simulink model "SSN_39busRT_Ctrl_4WT_19B"  (R2021a)
settings: Solver=ode3  StartTime=0.0  StopTime=10  FixedStep=Ts  MaxStep=1/60  RelTol=1e-2  AbsTol=1e-1
PreLoadFcn:
  | Ts=2.50e-6; ssn_ieee39_params; load('Pwf.mat');
InitFcn:
  | Ts=2.50e-6; ssn_ieee39_params; load('Pwf.mat');
values from neighbouring files (symbols this model uses):
  f = 50    [ssn_ieee39_params_ctrl.m]
  fNom = f    (= 60)    [ssn_ieee39_params_ctrl.m]
  ILR = 5.02    [ssn_ieee39_params_ctrl.m]
  IQMIN = 0.1    [ssn_ieee39_params_ctrl.m]
  ISCLIM = 1    [ssn_ieee39_params_ctrl.m]
  ITFpu = 1.10    (= 1.1)    [ssn_ieee39_params_ctrl.m]
  K = 1    [ssn_ieee39_params_ctrl.m]
  K1 = 1    [ssn_ieee39_params_ctrl.m]
  K2 = 2    [ssn_ieee39_params_ctrl.m]
  KCL = 1.04    [ssn_ieee39_params_ctrl.m]
  KFB = 0    [ssn_ieee39_params_ctrl.m]
  KFF = 1    [ssn_ieee39_params_ctrl.m]
  KFIX = 1    [ssn_ieee39_params_ctrl.m]
  KG = 1    [ssn_ieee39_params_ctrl.m]
  KIA = 59.91    [ssn_ieee39_params_ctrl.m]
  KIOEX = 0.0303    [ssn_ieee39_params_ctrl.m]
  KIUEX = 0.0303    [ssn_ieee39_params_ctrl.m]
  KIUOEX = 1    [ssn_ieee39_params_ctrl.m]
  KIUUEX = 1    [ssn_ieee39_params_ctrl.m]
  KLR = 22.47    [ssn_ieee39_params_ctrl.m]
  KM = 1    [ssn_ieee39_params_ctrl.m]
  KOEL = 0.24    [ssn_ieee39_params_ctrl.m]
  Kp = 1    [ssn_ieee39_params_ctrl.m]
  KPA = 30    [ssn_ieee39_params_ctrl.m]
  KPOEL = 1    [ssn_ieee39_params_ctrl.m]
  KPOEX = 0    [ssn_ieee39_params_ctrl.m]
  KPUEX = 0    [ssn_ieee39_params_ctrl.m]
  KSCALE = 0.319    [ssn_ieee39_params_ctrl.m]
  KUF = 0    [ssn_ieee39_params_ctrl.m]
  KUI = 0.001    [ssn_ieee39_params_ctrl.m]
  KUL = 0.24    [ssn_ieee39_params_ctrl.m]
  s = 10    [ssn_ieee39_params_ctrl.m]
  TA = 0.01    [ssn_ieee39_params_ctrl.m]
  Tadj = 0    [ssn_ieee39_params_ctrl.m]
  taps = [1 1 1.07 1.07 1.009 1.025 1 1.025 1.025 1.025]*1    [ssn_ieee39_params_ctrl.m]
  TF = 0.02    [ssn_ieee39_params_ctrl.m]
  TG = 0.024    [ssn_ieee39_params_ctrl.m]
  TINV = 0    [ssn_ieee39_params_ctrl.m]
  TIT = 0.1    [ssn_ieee39_params_ctrl.m]
  TL_10_11_len = 14    [ssn_ieee39_params_ctrl.m]
  TL_10_13_len = 14    [ssn_ieee39_params_ctrl.m]
  TL_13_14_len = 32    [ssn_ieee39_params_ctrl.m]
  TL_14_15_len = 70    [ssn_ieee39_params_ctrl.m]
  TL_15_16_len = 31.5    [ssn_ieee39_params_ctrl.m]
  TL_16_17_len = 26    [ssn_ieee39_params_ctrl.m]
  TL_16_19_len = 61    [ssn_ieee39_params_ctrl.m]
  TL_16_21_len = 46    [ssn_ieee39_params_ctrl.m]
  TL_16_24_len = 15    [ssn_ieee39_params_ctrl.m]
  TL_17_18_len = 26    [ssn_ieee39_params_ctrl.m]
  TL_17_27_len = 59    [ssn_ieee39_params_ctrl.m]
  TL_1_2_len = 134    [ssn_ieee39_params_ctrl.m]
  TL_1_39_len = 105    [ssn_ieee39_params_ctrl.m]
  TL_21_22_len = 47    [ssn_ieee39_params_ctrl.m]
  TL_22_23_len = 33    [ssn_ieee39_params_ctrl.m]
  TL_24_23_len = 88    [ssn_ieee39_params_ctrl.m]
  TL_25_26_len = 101    [ssn_ieee39_params_ctrl.m]
  TL_26_27_len = 46.5    [ssn_ieee39_params_ctrl.m]
  TL_26_28_len = 151    [ssn_ieee39_params_ctrl.m]
  TL_26_29_len = 200    [ssn_ieee39_params_ctrl.m]
  TL_28_29_len = 48    [ssn_ieee39_params_ctrl.m]
  TL_2_25_len = 28    [ssn_ieee39_params_ctrl.m]
  TL_2_2_len = 49    [ssn_ieee39_params_ctrl.m]
  TL_3_18_len = 42    [ssn_ieee39_params_ctrl.m]
  TL_3_4_len = 53    [ssn_ieee39_params_ctrl.m]
  TL_4_14_len = 33    [ssn_ieee39_params_ctrl.m]
  TL_4_5_len = 32.5    [ssn_ieee39_params_ctrl.m]
  TL_5_6_len = 14    [ssn_ieee39_params_ctrl.m]
  TL_5_8_len = 32    [ssn_ieee39_params_ctrl.m]
  TL_6_11_len = 26.5    [ssn_ieee39_params_ctrl.m]
  TL_6_7_len = 25.5    [ssn_ieee39_params_ctrl.m]
  TL_7_8_len = 15    [ssn_ieee39_params_ctrl.m]
  TL_8_9_len = 93    [ssn_ieee39_params_ctrl.m]
  TL_9_39_len = 136    [ssn_ieee39_params_ctrl.m]
  TOEL = 5.00    (= 5)    [ssn_ieee39_params_ctrl.m]
  TQREF = 0    [ssn_ieee39_params_ctrl.m]
  TQSCL = 0.012    [ssn_ieee39_params_ctrl.m]
  Ts_PMU = 1/1000    (= 0.001)    [ssn_ieee39_params_ctrl.m]
  TU1 = 0    [ssn_ieee39_params_ctrl.m]
  TU2 = 0    [ssn_ieee39_params_ctrl.m]
  TU3 = 0    [ssn_ieee39_params_ctrl.m]
  TU4 = 0    [ssn_ieee39_params_ctrl.m]
  TUL = 0    [ssn_ieee39_params_ctrl.m]
  TUP = 0.050    (= 0.05)    [ssn_ieee39_params_ctrl.m]
  TUQ = .005    (= 0.005)    [ssn_ieee39_params_ctrl.m]
  TUV = 0.2    [ssn_ieee39_params_ctrl.m]
  VAAMAX = VAMAX    (= 7.05)    [ssn_ieee39_params_ctrl.m]
  VAMAX = 7.05    [ssn_ieee39_params_ctrl.m]
  VAMIN = -6.11    [ssn_ieee39_params_ctrl.m]
  VBMAX = 999    [ssn_ieee39_params_ctrl.m]
  VF = 0    [ssn_ieee39_params_ctrl.m]
  VFB = 0    [ssn_ieee39_params_ctrl.m]
  VMMAX = 7.05    [ssn_ieee39_params_ctrl.m]
  VMMIN = -6.11    [ssn_ieee39_params_ctrl.m]
  VOELmax1 = 0.2353    [ssn_ieee39_params_ctrl.m]
  VOELmax2 = 0.0    (= 0)    [ssn_ieee39_params_ctrl.m]
  VOELmin1 = -0.24    [ssn_ieee39_params_ctrl.m]
  VOELmin2 = -1.0    (= -1)    [ssn_ieee39_params_ctrl.m]
  VRMAX = 7.05    [ssn_ieee39_params_ctrl.m]
  VRMIN = -6.11    [ssn_ieee39_params_ctrl.m]
  VSCLmax = 0.20    (= 0.2)    [ssn_ieee39_params_ctrl.m]
  VSCLmin = -0.10    (= -0.1)    [ssn_ieee39_params_ctrl.m]
  VUELmax1 = 1    [ssn_ieee39_params_ctrl.m]
  VUELmax2 = 1    [ssn_ieee39_params_ctrl.m]
  VUELmin1 = -1    [ssn_ieee39_params_ctrl.m]
  VUELmin2 = -1    [ssn_ieee39_params_ctrl.m]
  VUImax = 1    [ssn_ieee39_params_ctrl.m]
  VUImin = -1    [ssn_ieee39_params_ctrl.m]
undefined symbols (not defined in the file or in its folder): another_event_name, D1, Delta, DiscIntNeverNeededParam, find_system, MOV_segment9, my_event_name, powergui, Pw1, Pw2, Pw3, Pw4, vNomHV
libraries: powerlib_extras x162, spsThreePhaseVIMeasurementLib x55, spsCurrentMeasurementLib x52, simulink_extras x44, slpidlib x40, op_dpl_lib x36, spsST2AModel x20, spsThreePhaseParallelRLCLoadLib x20, spsThreePhaseTransformerTwoWindingsLib x17, spsControlledVoltageSourceLib x16, spsVoltageMeasurementLib x12, spsSynchronousMachinepuStandardLib x10
(part 4 of 19)

== system SSN_39busRT_Ctrl_4WT_19B/SM_master/PMU_Vpos_60Hz7 ==
  abc : Inport  PortDimensions=3
  1 / sqrt of 2 : Gain  Gain=1/sqrt(2)  OutDataTypeStr=Inherit: Same as input  ParamDataTypeStr=Inherit: Same as input
  Cartesian to Polar : simulink_extras/Transformations/Cartesian to Polar
  Demux : Demux  Outputs=3
      settings: DisplayOption=none
  Discrete Mean value1 : powerlib_extras/Discrete Measurements/Discrete  Mean value  Freq=Freq  Vinit=Real_Init  Ts=Ts
      settings: SourceProductBaseCode=PS
  Discrete Mean value2 : powerlib_extras/Discrete Measurements/Discrete  Mean value  Freq=Freq  Vinit=Imag_Init  Ts=Ts
      settings: SourceProductBaseCode=PS
  Discrete Derivative : simulink/Discrete/Discrete Derivative  gainval=1.0  ICPrevScaledInput=0.0  OutMin=[]  OutMax=[]  OutDataType=fixdt(1, 16)  OutScaling=2^-10  DoSatur=off
  Gain : Gain  Gain=2*pi*Freq  SaturateOnIntegerOverflow=on  OutDataTypeStr=Inherit: Same as input  ParamDataTypeStr=Inherit: Same as input
  Mux : Mux  Inputs=2
  Rad->Deg. : Gain  Gain=180/pi  SaturateOnIntegerOverflow=on  OutDataTypeStr=Inherit: Same as input  ParamDataTypeStr=Inherit: Same as input
  Sum : Sum  Inputs=|++  OutDataTypeStr=Inherit: Same as first input
  Terminator : Terminator
  Trigonometric Function : Trigonometry
  Trigonometric Function1 : Trigonometry  Operator=cos
  abc_to_dq0 Transformation : powerlib_extras/Measurements/abc_to_dq0 Transformation
      settings: SourceProductBaseCode=PS
  fo : Constant  Value=2*pi*Freq
  t : DigitalClock  SampleTime=Ts
  Mag : Outport
  Phase : Outport  Port=2
  freq : Outport  Port=3
  dfdt : Outport  Port=4
  wires:
  Cartesian to Polar/2 -> Rad->Deg./1, Discrete Derivative/1
  Gain/1 -> Trigonometric Function1/1, Trigonometric Function/1
  t/1 -> Gain/1
  abc/1 -> abc_to_dq0 Transformation/1
  Mux/1 -> abc_to_dq0 Transformation/2
  Discrete Mean value1/1 -> Cartesian to Polar/1  "Real"
  Rad->Deg./1 -> Phase/1
  Discrete Mean value2/1 -> Cartesian to Polar/2  "Real"
  abc_to_dq0 Transformation/1 -> Demux/1
  Demux/3 -> Terminator/1
  Demux/2 -> Discrete Mean value2/1
  Demux/1 -> Discrete Mean value1/1
  Trigonometric Function/1 -> Mux/1
  Trigonometric Function1/1 -> Mux/2
  Cartesian to Polar/1 -> 1 / sqrt of 2/1
  1 / sqrt of 2/1 -> Mag/1
  Discrete Derivative/1 -> Sum/2, dfdt/1
  fo/1 -> Sum/1
  Sum/1 -> freq/1

== system SSN_39busRT_Ctrl_4WT_19B/SM_master/PMU_Vpos_60Hz8 ==
  abc : Inport  PortDimensions=3
  1 / sqrt of 2 : Gain  Gain=1/sqrt(2)  OutDataTypeStr=Inherit: Same as input  ParamDataTypeStr=Inherit: Same as input
  Cartesian to Polar : simulink_extras/Transformations/Cartesian to Polar
  Demux : Demux  Outputs=3
      settings: DisplayOption=none
  Discrete Mean value1 : powerlib_extras/Discrete Measurements/Discrete  Mean value  Freq=Freq  Vinit=Real_Init  Ts=Ts
      settings: SourceProductBaseCode=PS
  Discrete Mean value2 : powerlib_extras/Discrete Measurements/Discrete  Mean value  Freq=Freq  Vinit=Imag_Init  Ts=Ts
      settings: SourceProductBaseCode=PS
  Discrete Derivative : simulink/Discrete/Discrete Derivative  gainval=1.0  ICPrevScaledInput=0.0  OutMin=[]  OutMax=[]  OutDataType=fixdt(1, 16)  OutScaling=2^-10  DoSatur=off
  Gain : Gain  Gain=2*pi*Freq  SaturateOnIntegerOverflow=on  OutDataTypeStr=Inherit: Same as input  ParamDataTypeStr=Inherit: Same as input
  Mux : Mux  Inputs=2
  Rad->Deg. : Gain  Gain=180/pi  SaturateOnIntegerOverflow=on  OutDataTypeStr=Inherit: Same as input  ParamDataTypeStr=Inherit: Same as input
  Sum : Sum  Inputs=|++  OutDataTypeStr=Inherit: Same as first input
  Terminator : Terminator
  Trigonometric Function : Trigonometry
  Trigonometric Function1 : Trigonometry  Operator=cos
  abc_to_dq0 Transformation : powerlib_extras/Measurements/abc_to_dq0 Transformation
      settings: SourceProductBaseCode=PS
  fo : Constant  Value=2*pi*Freq
  t : DigitalClock  SampleTime=Ts
  Mag : Outport
  Phase : Outport  Port=2
  freq : Outport  Port=3
  dfdt : Outport  Port=4
  wires:
  Cartesian to Polar/2 -> Rad->Deg./1, Discrete Derivative/1
  Gain/1 -> Trigonometric Function1/1, Trigonometric Function/1
  t/1 -> Gain/1
  abc/1 -> abc_to_dq0 Transformation/1
  Mux/1 -> abc_to_dq0 Transformation/2
  Discrete Mean value1/1 -> Cartesian to Polar/1  "Real"
  Rad->Deg./1 -> Phase/1
  Discrete Mean value2/1 -> Cartesian to Polar/2  "Real"
  abc_to_dq0 Transformation/1 -> Demux/1
  Demux/3 -> Terminator/1
  Demux/2 -> Discrete Mean value2/1
  Demux/1 -> Discrete Mean value1/1
  Trigonometric Function/1 -> Mux/1
  Trigonometric Function1/1 -> Mux/2
  Cartesian to Polar/1 -> 1 / sqrt of 2/1
  1 / sqrt of 2/1 -> Mag/1
  Discrete Derivative/1 -> Sum/2, dfdt/1
  fo/1 -> Sum/1
  Sum/1 -> freq/1

== system SSN_39busRT_Ctrl_4WT_19B/SM_master/PMU_Vpos_60Hz9 ==
  abc : Inport  PortDimensions=3
  1 / sqrt of 2 : Gain  Gain=1/sqrt(2)  OutDataTypeStr=Inherit: Same as input  ParamDataTypeStr=Inherit: Same as input
  Cartesian to Polar : simulink_extras/Transformations/Cartesian to Polar
  Demux : Demux  Outputs=3
      settings: DisplayOption=none
  Discrete Mean value1 : powerlib_extras/Discrete Measurements/Discrete  Mean value  Freq=Freq  Vinit=Real_Init  Ts=Ts
      settings: SourceProductBaseCode=PS
  Discrete Mean value2 : powerlib_extras/Discrete Measurements/Discrete  Mean value  Freq=Freq  Vinit=Imag_Init  Ts=Ts
      settings: SourceProductBaseCode=PS
  Discrete Derivative : simulink/Discrete/Discrete Derivative  gainval=1.0  ICPrevScaledInput=0.0  OutMin=[]  OutMax=[]  OutDataType=fixdt(1, 16)  OutScaling=2^-10  DoSatur=off
  Gain : Gain  Gain=2*pi*Freq  SaturateOnIntegerOverflow=on  OutDataTypeStr=Inherit: Same as input  ParamDataTypeStr=Inherit: Same as input
  Mux : Mux  Inputs=2
  Rad->Deg. : Gain  Gain=180/pi  SaturateOnIntegerOverflow=on  OutDataTypeStr=Inherit: Same as input  ParamDataTypeStr=Inherit: Same as input
  Sum : Sum  Inputs=|++  OutDataTypeStr=Inherit: Same as first input
  Terminator : Terminator
  Trigonometric Function : Trigonometry
  Trigonometric Function1 : Trigonometry  Operator=cos
  abc_to_dq0 Transformation : powerlib_extras/Measurements/abc_to_dq0 Transformation
      settings: SourceProductBaseCode=PS
  fo : Constant  Value=2*pi*Freq
  t : DigitalClock  SampleTime=Ts
  Mag : Outport
  Phase : Outport  Port=2
  freq : Outport  Port=3
  dfdt : Outport  Port=4
  wires:
  Cartesian to Polar/2 -> Rad->Deg./1, Discrete Derivative/1
  Gain/1 -> Trigonometric Function1/1, Trigonometric Function/1
  t/1 -> Gain/1
  abc/1 -> abc_to_dq0 Transformation/1
  Mux/1 -> abc_to_dq0 Transformation/2
  Discrete Mean value1/1 -> Cartesian to Polar/1  "Real"
  Rad->Deg./1 -> Phase/1
  Discrete Mean value2/1 -> Cartesian to Polar/2  "Real"
  abc_to_dq0 Transformation/1 -> Demux/1
  Demux/3 -> Terminator/1
  Demux/2 -> Discrete Mean value2/1
  Demux/1 -> Discrete Mean value1/1
  Trigonometric Function/1 -> Mux/1
  Trigonometric Function1/1 -> Mux/2
  Cartesian to Polar/1 -> 1 / sqrt of 2/1
  1 / sqrt of 2/1 -> Mag/1
  Discrete Derivative/1 -> Sum/2, dfdt/1
  fo/1 -> Sum/1
  Sum/1 -> freq/1

== system SSN_39busRT_Ctrl_4WT_19B/SM_master/Power ==
  Mux : Mux  Inputs=10
  Power (3ph, Instantaneous){1..10} (10 alike) : spsPower3phInstantaneousLib/Power (3ph, Instantaneous)
  Scope{1..10} (10 alike) : Scope  NumInputPorts=2
  to PU{1..20} (20 alike) : Gain
  Pgen : Outport
  tag scope: PG_10=global, PG_1=global, PG_2=global, PG_3=global, PG_4=global, PG_5=global, PG_6=global, PG_7=global, PG_8=global, PG_9=global
  wires:
  [Iabc_30] -> "Power (3ph, Instantaneous)1"/2
  to PU2/1 -> Scope7/2, [QG_10]
  [Vabc_30] -> "Power (3ph, Instantaneous)1"/1
  "Power (3ph, Instantaneous)4"/2 -> to PU9/1
  to PU8/1 -> [PG_8], Scope4/1
  "Power (3ph, Instantaneous)1"/1 -> to PU1/1
  "Power (3ph, Instantaneous)1"/2 -> to PU2/1
  "Power (3ph, Instantaneous)4"/1 -> to PU8/1
  [Vabc_37] -> "Power (3ph, Instantaneous)4"/1
  to PU1/1 -> Scope7/1, [PG_10]
  [Iabc_37] -> "Power (3ph, Instantaneous)4"/2
  to PU9/1 -> [QG_8], Scope4/2
  to PU6/1 -> Scope1/2, [QG_9]
  [Iabc_38] -> "Power (3ph, Instantaneous)3"/2
  to PU3/1 -> [PG_1], Scope2/1
  [Vabc_38] -> "Power (3ph, Instantaneous)3"/1
  "Power (3ph, Instantaneous)3"/1 -> to PU5/1
  "Power (3ph, Instantaneous)2"/2 -> to PU4/1
  "Power (3ph, Instantaneous)2"/1 -> to PU3/1
  to PU5/1 -> Scope1/1, [PG_9]
  "Power (3ph, Instantaneous)3"/2 -> to PU6/1
  [Vabc_391] -> "Power (3ph, Instantaneous)2"/1
  to PU4/1 -> [QG_1], Scope2/2
  [Iabc_391] -> "Power (3ph, Instantaneous)2"/2
  [Iabc_34] -> "Power (3ph, Instantaneous)6"/2
  to PU12/1 -> Scope5/2, [QG_5]
  [Vabc_34] -> "Power (3ph, Instantaneous)6"/1
  "Power (3ph, Instantaneous)7"/2 -> to PU14/1
  to PU13/1 -> [PG_4], Scope3/1
  "Power (3ph, Instantaneous)6"/1 -> to PU11/1
  "Power (3ph, Instantaneous)6"/2 -> to PU12/1
  "Power (3ph, Instantaneous)7"/1 -> to PU13/1
  [Vabc_33] -> "Power (3ph, Instantaneous)7"/1
  to PU11/1 -> Scope5/1, [PG_5]
  [Iabc_33] -> "Power (3ph, Instantaneous)7"/2
  to PU14/1 -> [QG_4], Scope3/2
  to PU16/1 -> Scope6/2, [QG_2]
  [Iabc_31] -> "Power (3ph, Instantaneous)8"/2
  to PU7/1 -> [PG_3], Scope8/1
  [Vabc_31] -> "Power (3ph, Instantaneous)8"/1
  "Power (3ph, Instantaneous)8"/1 -> to PU15/1
  "Power (3ph, Instantaneous)5"/2 -> to PU10/1
  "Power (3ph, Instantaneous)5"/1 -> to PU7/1
  to PU15/1 -> Scope6/1, [PG_2]
  "Power (3ph, Instantaneous)8"/2 -> to PU16/1
  [Vabc_32] -> "Power (3ph, Instantaneous)5"/1
  to PU10/1 -> [QG_3], Scope8/2
  [Iabc_32] -> "Power (3ph, Instantaneous)5"/2
  [Iabc_35] -> "Power (3ph, Instantaneous)9"/2
  to PU17/1 -> Scope10/2, [QG_6]
  [Vabc_35] -> "Power (3ph, Instantaneous)9"/1
  "Power (3ph, Instantaneous)9"/1 -> to PU20/1
  "Power (3ph, Instantaneous)9"/2 -> to PU17/1
  to PU20/1 -> Scope10/1, [PG_6]
  to PU18/1 -> [PG_7], Scope9/1
  "Power (3ph, Instantaneous)10"/2 -> to PU19/1
  "Power (3ph, Instantaneous)10"/1 -> to PU18/1
  [Vabc_36] -> "Power (3ph, Instantaneous)10"/1
  to PU19/1 -> [QG_7], Scope9/2
  [Iabc_36] -> "Power (3ph, Instantaneous)10"/2
  [PG_1] -> Mux/1
  [PG_2] -> Mux/2
  [PG_3] -> Mux/3
  [PG_4] -> Mux/4
  [PG_5] -> Mux/5
  [PG_6] -> Mux/6
  [PG_7] -> Mux/7
  [PG_8] -> Mux/8
  [PG_9] -> Mux/9
  [PG_10] -> Mux/10
  Mux/1 -> Pgen/1

== system SSN_39busRT_Ctrl_4WT_19B/powergui/EquivalentModel1 ==
  Sources : Subsystem
  State-Space : S-Function  FunctionName=ssn_sfun_v1  Parameters=1,0  SFunctionDeploymentMode=off  EnableBusSupport=off  SFcnStateName=MOV_segment9,MOV_segment9,MOV_segment9,MOV_segment9,MOV_segment9,MOV_segment9,MOV_segment9,MOV_segment9,MOV_segment9,MOV_segment9
      settings: SFcnIsStateOwnerBlock=on
  Yout : Subsystem
  wires:
  State-Space/1 -> Yout/1(v,i)
  Sources/1(u) -> State-Space/1

== system SSN_39busRT_Ctrl_4WT_19B/powergui/EquivalentModel10 ==
  Sources : Subsystem
  State-Space : S-Function  FunctionName=ssn_sfun_v1  Parameters=10,0  SFunctionDeploymentMode=off  EnableBusSupport=off  SFcnStateName=MOV_segment9,MOV_segment9,MOV_segment9,MOV_segment9,MOV_segment9,MOV_segment9,MOV_segment9,MOV_segment9,MOV_segment9,MOV_segment9
      settings: SFcnIsStateOwnerBlock=on
  Yout : Subsystem
  wires:
  State-Space/1 -> Yout/1(v,i)
  Sources/1(u) -> State-Space/1

== system SSN_39busRT_Ctrl_4WT_19B/powergui/EquivalentModel11 ==
  Sources : Subsystem
  State-Space : S-Function  FunctionName=ssn_sfun_v1  Parameters=11,0  SFunctionDeploymentMode=off  EnableBusSupport=off  SFcnStateName=MOV_segment9,MOV_segment9,MOV_segment9,MOV_segment9,MOV_segment9,MOV_segment9,MOV_segment9,MOV_segment9,MOV_segment9,MOV_segment9
      settings: SFcnIsStateOwnerBlock=on
  Yout : Subsystem
  wires:
  State-Space/1 -> Yout/1(v,i)
  Sources/1(u) -> State-Space/1

== system SSN_39busRT_Ctrl_4WT_19B/powergui/EquivalentModel12 ==
  Sources : Subsystem
  State-Space : S-Function  FunctionName=ssn_sfun_v1  Parameters=12,0  SFunctionDeploymentMode=off  EnableBusSupport=off  SFcnStateName=MOV_segment9,MOV_segment9,MOV_segment9,MOV_segment9,MOV_segment9,MOV_segment9,MOV_segment9,MOV_segment9,MOV_segment9,MOV_segment9
      settings: SFcnIsStateOwnerBlock=on
  Yout : Subsystem
  wires:
  State-Space/1 -> Yout/1(v,i)
  Sources/1(u) -> State-Space/1

== system SSN_39busRT_Ctrl_4WT_19B/powergui/EquivalentModel13 ==
  Sources : Subsystem
  State-Space : S-Function  FunctionName=ssn_sfun_v1  Parameters=13,0  SFunctionDeploymentMode=off  EnableBusSupport=off  SFcnStateName=MOV_segment9,MOV_segment9,MOV_segment9,MOV_segment9,MOV_segment9,MOV_segment9,MOV_segment9,MOV_segment9,MOV_segment9,MOV_segment9
      settings: SFcnIsStateOwnerBlock=on
  Yout : Subsystem
  wires:
  State-Space/1 -> Yout/1(v,i)
  Sources/1(u) -> State-Space/1

== system SSN_39busRT_Ctrl_4WT_19B/powergui/EquivalentModel14 ==
  Sources : Subsystem
  State-Space : S-Function  FunctionName=ssn_sfun_v1  Parameters=14,0  SFunctionDeploymentMode=off  EnableBusSupport=off  SFcnStateName=MOV_segment9,MOV_segment9,MOV_segment9,MOV_segment9,MOV_segment9,MOV_segment9,MOV_segment9,MOV_segment9,MOV_segment9,MOV_segment9
      settings: SFcnIsStateOwnerBlock=on
  Yout : Subsystem
  wires:
  State-Space/1 -> Yout/1(v,i)
  Sources/1(u) -> State-Space/1

== system SSN_39busRT_Ctrl_4WT_19B/powergui/EquivalentModel15 ==
  Sources : Subsystem
  State-Space : S-Function  FunctionName=ssn_sfun_v1  Parameters=15,0  SFunctionDeploymentMode=off  EnableBusSupport=off  SFcnStateName=MOV_segment9,MOV_segment9,MOV_segment9,MOV_segment9,MOV_segment9,MOV_segment9,MOV_segment9,MOV_segment9,MOV_segment9,MOV_segment9
      settings: SFcnIsStateOwnerBlock=on
  Yout : Subsystem
  wires:
  State-Space/1 -> Yout/1(v,i)
  Sources/1(u) -> State-Space/1

== system SSN_39busRT_Ctrl_4WT_19B/powergui/EquivalentModel16 ==
  Gates : Subsystem
  Sources : Subsystem
  State-Space : S-Function  FunctionName=ssn_sfun_v1  Parameters=16,0  SFunctionDeploymentMode=off  EnableBusSupport=off  SFcnStateName=MOV_segment9,MOV_segment9,MOV_segment9,MOV_segment9,MOV_segment9,MOV_segment9,MOV_segment9,MOV_segment9,MOV_segment9,MOV_segment9
      settings: SFcnIsStateOwnerBlock=on
  Status : Subsystem
  Yout : Subsystem
  wires:
  Gates/1(gates) -> State-Space/2
  Sources/1(u) -> State-Space/1
  State-Space/2 -> Status/1(status)
  State-Space/1 -> Yout/1(v,i)

== system SSN_39busRT_Ctrl_4WT_19B/powergui/EquivalentModel17 ==
  Sources : Subsystem
  State-Space : S-Function  FunctionName=ssn_sfun_v1  Parameters=17,0  SFunctionDeploymentMode=off  EnableBusSupport=off  SFcnStateName=MOV_segment9,MOV_segment9,MOV_segment9,MOV_segment9,MOV_segment9,MOV_segment9,MOV_segment9,MOV_segment9,MOV_segment9,MOV_segment9
      settings: SFcnIsStateOwnerBlock=on
  Yout : Subsystem
  wires:
  State-Space/1 -> Yout/1(v,i)
  Sources/1(u) -> State-Space/1

== system SSN_39busRT_Ctrl_4WT_19B/powergui/EquivalentModel18 ==
  Sources : Subsystem
  State-Space : S-Function  FunctionName=ssn_sfun_v1  Parameters=18,0  SFunctionDeploymentMode=off  EnableBusSupport=off  SFcnStateName=MOV_segment9,MOV_segment9,MOV_segment9,MOV_segment9,MOV_segment9,MOV_segment9,MOV_segment9,MOV_segment9,MOV_segment9,MOV_segment9
      settings: SFcnIsStateOwnerBlock=on
  Yout : Subsystem
  wires:
  State-Space/1 -> Yout/1(v,i)
  Sources/1(u) -> State-Space/1

== system SSN_39busRT_Ctrl_4WT_19B/powergui/EquivalentModel19 ==
  Sources : Subsystem
  State-Space : S-Function  FunctionName=ssn_sfun_v1  Parameters=19,0  SFunctionDeploymentMode=off  EnableBusSupport=off  SFcnStateName=MOV_segment9,MOV_segment9,MOV_segment9,MOV_segment9,MOV_segment9,MOV_segment9,MOV_segment9,MOV_segment9,MOV_segment9,MOV_segment9
      settings: SFcnIsStateOwnerBlock=on
  Yout : Subsystem
  wires:
  State-Space/1 -> Yout/1(v,i)
  Sources/1(u) -> State-Space/1

== system SSN_39busRT_Ctrl_4WT_19B/powergui/EquivalentModel2 ==
  Sources : Subsystem
  State-Space : S-Function  FunctionName=ssn_sfun_v1  Parameters=2,0  SFunctionDeploymentMode=off  EnableBusSupport=off  SFcnStateName=MOV_segment9,MOV_segment9,MOV_segment9,MOV_segment9,MOV_segment9,MOV_segment9,MOV_segment9,MOV_segment9,MOV_segment9,MOV_segment9
      settings: SFcnIsStateOwnerBlock=on
  Yout : Subsystem
  wires:
  State-Space/1 -> Yout/1(v,i)
  Sources/1(u) -> State-Space/1

== system SSN_39busRT_Ctrl_4WT_19B/powergui/EquivalentModel20 ==
  Sources : Subsystem
  State-Space : S-Function  FunctionName=ssn_sfun_v1  Parameters=20,0  SFunctionDeploymentMode=off  EnableBusSupport=off  SFcnStateName=MOV_segment9,MOV_segment9,MOV_segment9,MOV_segment9,MOV_segment9,MOV_segment9,MOV_segment9,MOV_segment9,MOV_segment9,MOV_segment9
      settings: SFcnIsStateOwnerBlock=on
  Yout : Subsystem
  wires:
  State-Space/1 -> Yout/1(v,i)
  Sources/1(u) -> State-Space/1

== system SSN_39busRT_Ctrl_4WT_19B/powergui/EquivalentModel21 ==
  Sources : Subsystem
  State-Space : S-Function  FunctionName=ssn_sfun_v1  Parameters=21,0  SFunctionDeploymentMode=off  EnableBusSupport=off  SFcnStateName=MOV_segment9,MOV_segment9,MOV_segment9,MOV_segment9,MOV_segment9,MOV_segment9,MOV_segment9,MOV_segment9,MOV_segment9,MOV_segment9
      settings: SFcnIsStateOwnerBlock=on
  Yout : Subsystem
  wires:
  State-Space/1 -> Yout/1(v,i)
  Sources/1(u) -> State-Space/1

== system SSN_39busRT_Ctrl_4WT_19B/powergui/EquivalentModel22 ==
  Sources : Subsystem
  State-Space : S-Function  FunctionName=ssn_sfun_v1  Parameters=22,0  SFunctionDeploymentMode=off  EnableBusSupport=off  SFcnStateName=MOV_segment9,MOV_segment9,MOV_segment9,MOV_segment9,MOV_segment9,MOV_segment9,MOV_segment9,MOV_segment9,MOV_segment9,MOV_segment9
      settings: SFcnIsStateOwnerBlock=on
  Yout : Subsystem
  wires:
  State-Space/1 -> Yout/1(v,i)
  Sources/1(u) -> State-Space/1

== system SSN_39busRT_Ctrl_4WT_19B/powergui/EquivalentModel23 ==
  Sources : Subsystem
  State-Space : S-Function  FunctionName=ssn_sfun_v1  Parameters=23,0  SFunctionDeploymentMode=off  EnableBusSupport=off  SFcnStateName=MOV_segment9,MOV_segment9,MOV_segment9,MOV_segment9,MOV_segment9,MOV_segment9,MOV_segment9,MOV_segment9,MOV_segment9,MOV_segment9
      settings: SFcnIsStateOwnerBlock=on
  Yout : Subsystem
  wires:
  State-Space/1 -> Yout/1(v,i)
  Sources/1(u) -> State-Space/1

== system SSN_39busRT_Ctrl_4WT_19B/powergui/EquivalentModel24 ==
  Sources : Subsystem
  State-Space : S-Function  FunctionName=ssn_sfun_v1  Parameters=24,0  SFunctionDeploymentMode=off  EnableBusSupport=off  SFcnStateName=MOV_segment9,MOV_segment9,MOV_segment9,MOV_segment9,MOV_segment9,MOV_segment9,MOV_segment9,MOV_segment9,MOV_segment9,MOV_segment9
      settings: SFcnIsStateOwnerBlock=on
  Yout : Subsystem
  wires:
  State-Space/1 -> Yout/1(v,i)
  Sources/1(u) -> State-Space/1

== system SSN_39busRT_Ctrl_4WT_19B/powergui/EquivalentModel25 ==
  Sources : Subsystem
  State-Space : S-Function  FunctionName=ssn_sfun_v1  Parameters=25,0  SFunctionDeploymentMode=off  EnableBusSupport=off  SFcnStateName=MOV_segment9,MOV_segment9,MOV_segment9,MOV_segment9,MOV_segment9,MOV_segment9,MOV_segment9,MOV_segment9,MOV_segment9,MOV_segment9
      settings: SFcnIsStateOwnerBlock=on
  Yout : Subsystem
  wires:
  State-Space/1 -> Yout/1(v,i)
  Sources/1(u) -> State-Space/1

== system SSN_39busRT_Ctrl_4WT_19B/powergui/EquivalentModel26 ==
  Sources : Subsystem
  State-Space : S-Function  FunctionName=ssn_sfun_v1  Parameters=26,0  SFunctionDeploymentMode=off  EnableBusSupport=off  SFcnStateName=MOV_segment9,MOV_segment9,MOV_segment9,MOV_segment9,MOV_segment9,MOV_segment9,MOV_segment9,MOV_segment9,MOV_segment9,MOV_segment9
      settings: SFcnIsStateOwnerBlock=on
  Yout : Subsystem
  wires:
  State-Space/1 -> Yout/1(v,i)
  Sources/1(u) -> State-Space/1

== system SSN_39busRT_Ctrl_4WT_19B/powergui/EquivalentModel27 ==
  Sources : Subsystem
  State-Space : S-Function  FunctionName=ssn_sfun_v1  Parameters=27,0  SFunctionDeploymentMode=off  EnableBusSupport=off  SFcnStateName=MOV_segment9,MOV_segment9,MOV_segment9,MOV_segment9,MOV_segment9,MOV_segment9,MOV_segment9,MOV_segment9,MOV_segment9,MOV_segment9
      settings: SFcnIsStateOwnerBlock=on
  Yout : Subsystem
  wires:
  State-Space/1 -> Yout/1(v,i)
  Sources/1(u) -> State-Space/1

== system SSN_39busRT_Ctrl_4WT_19B/powergui/EquivalentModel28 ==
  Sources : Subsystem
  State-Space : S-Function  FunctionName=ssn_sfun_v1  Parameters=28,0  SFunctionDeploymentMode=off  EnableBusSupport=off  SFcnStateName=MOV_segment9,MOV_segment9,MOV_segment9,MOV_segment9,MOV_segment9,MOV_segment9,MOV_segment9,MOV_segment9,MOV_segment9,MOV_segment9
      settings: SFcnIsStateOwnerBlock=on
  Yout : Subsystem
  wires:
  State-Space/1 -> Yout/1(v,i)
  Sources/1(u) -> State-Space/1

== system SSN_39busRT_Ctrl_4WT_19B/powergui/EquivalentModel29 ==
  Sources : Subsystem
  State-Space : S-Function  FunctionName=ssn_sfun_v1  Parameters=29,0  SFunctionDeploymentMode=off  EnableBusSupport=off  SFcnStateName=MOV_segment9,MOV_segment9,MOV_segment9,MOV_segment9,MOV_segment9,MOV_segment9,MOV_segment9,MOV_segment9,MOV_segment9,MOV_segment9
      settings: SFcnIsStateOwnerBlock=on
  Yout : Subsystem
  wires:
  State-Space/1 -> Yout/1(v,i)
  Sources/1(u) -> State-Space/1

== system SSN_39busRT_Ctrl_4WT_19B/powergui/EquivalentModel3 ==
  Sources : Subsystem
  State-Space : S-Function  FunctionName=ssn_sfun_v1  Parameters=3,0  SFunctionDeploymentMode=off  EnableBusSupport=off  SFcnStateName=MOV_segment9,MOV_segment9,MOV_segment9,MOV_segment9,MOV_segment9,MOV_segment9,MOV_segment9,MOV_segment9,MOV_segment9,MOV_segment9
      settings: SFcnIsStateOwnerBlock=on
  Yout : Subsystem
  wires:
  State-Space/1 -> Yout/1(v,i)
  Sources/1(u) -> State-Space/1

== system SSN_39busRT_Ctrl_4WT_19B/powergui/EquivalentModel30 ==
  Sources : Subsystem
  State-Space : S-Function  FunctionName=ssn_sfun_v1  Parameters=30,0  SFunctionDeploymentMode=off  EnableBusSupport=off  SFcnStateName=MOV_segment9,MOV_segment9,MOV_segment9,MOV_segment9,MOV_segment9,MOV_segment9,MOV_segment9,MOV_segment9,MOV_segment9,MOV_segment9
      settings: SFcnIsStateOwnerBlock=on
  Yout : Subsystem
  wires:
  State-Space/1 -> Yout/1(v,i)
  Sources/1(u) -> State-Space/1

== system SSN_39busRT_Ctrl_4WT_19B/powergui/EquivalentModel31 ==
  Sources : Subsystem
  State-Space : S-Function  FunctionName=ssn_sfun_v1  Parameters=31,0  SFunctionDeploymentMode=off  EnableBusSupport=off  SFcnStateName=MOV_segment9,MOV_segment9,MOV_segment9,MOV_segment9,MOV_segment9,MOV_segment9,MOV_segment9,MOV_segment9,MOV_segment9,MOV_segment9
      settings: SFcnIsStateOwnerBlock=on
  Yout : Subsystem
  wires:
  State-Space/1 -> Yout/1(v,i)
  Sources/1(u) -> State-Space/1

== system SSN_39busRT_Ctrl_4WT_19B/powergui/EquivalentModel32 ==
  Sources : Subsystem
  State-Space : S-Function  FunctionName=ssn_sfun_v1  Parameters=32,0  SFunctionDeploymentMode=off  EnableBusSupport=off  SFcnStateName=MOV_segment9,MOV_segment9,MOV_segment9,MOV_segment9,MOV_segment9,MOV_segment9,MOV_segment9,MOV_segment9,MOV_segment9,MOV_segment9
      settings: SFcnIsStateOwnerBlock=on
  Yout : Subsystem
  wires:
  State-Space/1 -> Yout/1(v,i)
  Sources/1(u) -> State-Space/1

== system SSN_39busRT_Ctrl_4WT_19B/powergui/EquivalentModel33 ==
  Sources : Subsystem
  State-Space : S-Function  FunctionName=ssn_sfun_v1  Parameters=33,0  SFunctionDeploymentMode=off  EnableBusSupport=off  SFcnStateName=MOV_segment9,MOV_segment9,MOV_segment9,MOV_segment9,MOV_segment9,MOV_segment9,MOV_segment9,MOV_segment9,MOV_segment9,MOV_segment9
      settings: SFcnIsStateOwnerBlock=on
  Yout : Subsystem
  wires:
  State-Space/1 -> Yout/1(v,i)
  Sources/1(u) -> State-Space/1

== system SSN_39busRT_Ctrl_4WT_19B/powergui/EquivalentModel34 ==
  Sources : Subsystem
  State-Space : S-Function  FunctionName=ssn_sfun_v1  Parameters=34,0  SFunctionDeploymentMode=off  EnableBusSupport=off  SFcnStateName=MOV_segment9,MOV_segment9,MOV_segment9,MOV_segment9,MOV_segment9,MOV_segment9,MOV_segment9,MOV_segment9,MOV_segment9,MOV_segment9
      settings: SFcnIsStateOwnerBlock=on
  Yout : Subsystem
  wires:
  State-Space/1 -> Yout/1(v,i)
  Sources/1(u) -> State-Space/1

== system SSN_39busRT_Ctrl_4WT_19B/powergui/EquivalentModel4 ==
  Sources : Subsystem
  State-Space : S-Function  FunctionName=ssn_sfun_v1  Parameters=4,0  SFunctionDeploymentMode=off  EnableBusSupport=off  SFcnStateName=MOV_segment9,MOV_segment9,MOV_segment9,MOV_segment9,MOV_segment9,MOV_segment9,MOV_segment9,MOV_segment9,MOV_segment9,MOV_segment9
      settings: SFcnIsStateOwnerBlock=on
  Yout : Subsystem
  wires:
  State-Space/1 -> Yout/1(v,i)
  Sources/1(u) -> State-Space/1

== system SSN_39busRT_Ctrl_4WT_19B/powergui/EquivalentModel5 ==
  Sources : Subsystem
  State-Space : S-Function  FunctionName=ssn_sfun_v1  Parameters=5,0  SFunctionDeploymentMode=off  EnableBusSupport=off  SFcnStateName=MOV_segment9,MOV_segment9,MOV_segment9,MOV_segment9,MOV_segment9,MOV_segment9,MOV_segment9,MOV_segment9,MOV_segment9,MOV_segment9
      settings: SFcnIsStateOwnerBlock=on
  Yout : Subsystem
  wires:
  State-Space/1 -> Yout/1(v,i)
  Sources/1(u) -> State-Space/1

== system SSN_39busRT_Ctrl_4WT_19B/powergui/EquivalentModel6 ==
  Sources : Subsystem
  State-Space : S-Function  FunctionName=ssn_sfun_v1  Parameters=6,0  SFunctionDeploymentMode=off  EnableBusSupport=off  SFcnStateName=MOV_segment9,MOV_segment9,MOV_segment9,MOV_segment9,MOV_segment9,MOV_segment9,MOV_segment9,MOV_segment9,MOV_segment9,MOV_segment9
      settings: SFcnIsStateOwnerBlock=on
  Yout : Subsystem
  wires:
  State-Space/1 -> Yout/1(v,i)
  Sources/1(u) -> State-Space/1

== system SSN_39busRT_Ctrl_4WT_19B/powergui/EquivalentModel7 ==
  Sources : Subsystem
  State-Space : S-Function  FunctionName=ssn_sfun_v1  Parameters=7,0  SFunctionDeploymentMode=off  EnableBusSupport=off  SFcnStateName=MOV_segment9,MOV_segment9,MOV_segment9,MOV_segment9,MOV_segment9,MOV_segment9,MOV_segment9,MOV_segment9,MOV_segment9,MOV_segment9
      settings: SFcnIsStateOwnerBlock=on
  Yout : Subsystem
  wires:
  State-Space/1 -> Yout/1(v,i)
  Sources/1(u) -> State-Space/1

== system SSN_39busRT_Ctrl_4WT_19B/powergui/EquivalentModel8 ==
  Sources : Subsystem
  State-Space : S-Function  FunctionName=ssn_sfun_v1  Parameters=8,0  SFunctionDeploymentMode=off  EnableBusSupport=off  SFcnStateName=MOV_segment9,MOV_segment9,MOV_segment9,MOV_segment9,MOV_segment9,MOV_segment9,MOV_segment9,MOV_segment9,MOV_segment9,MOV_segment9
      settings: SFcnIsStateOwnerBlock=on
  Yout : Subsystem
  wires:
  State-Space/1 -> Yout/1(v,i)
  Sources/1(u) -> State-Space/1

== system SSN_39busRT_Ctrl_4WT_19B/powergui/EquivalentModel9 ==
  Sources : Subsystem
  State-Space : S-Function  FunctionName=ssn_sfun_v1  Parameters=9,0  SFunctionDeploymentMode=off  EnableBusSupport=off  SFcnStateName=MOV_segment9,MOV_segment9,MOV_segment9,MOV_segment9,MOV_segment9,MOV_segment9,MOV_segment9,MOV_segment9,MOV_segment9,MOV_segment9
      settings: SFcnIsStateOwnerBlock=on
  Yout : Subsystem
  wires:
  State-Space/1 -> Yout/1(v,i)
  Sources/1(u) -> State-Space/1

== system SSN_39busRT_Ctrl_4WT_19B/SM_master/4 WT/SS_windfarm1to2 ==
  Ctrl_wf12 : Inport
  Bus Creator1 : BusCreator  Inputs=3
  Demux : Demux  Outputs=[2 2]
  Demux1 : Demux  Outputs=[1 1]
  Demux2 : Demux  Outputs=[1 1]
  Memory2 : Memory
  OpComm : rtlab/OpComm  nbport=1  groupe_acq=1  subsys_rate=Ts_grid  st=Ts_grid  Synchronization=on  Interpolation=on  Threshold=1.0  Missed_Data=off  Sim_Time=off  Samples=off  dynSigOut=off  from_console=0  warning_done=off  writeOpCommFile=off  Offset=off
      settings: SourceProductName=RT-LAB
  Simulation monitoring1 : Subsystem
  Terminator : Terminator
  Terminator1 : Terminator
  Wind Farm (DFIG Type) : Subsystem  mask(Wind Farm (DFIG Type)){fNom=fNom, vNom=1.025*vNomHV*(1E-3), Nwt=200, vMin=[0.5, 0.88], vMax=|, tTripV=[0.24  4.8  0.24], fMin=fNom-0.7, fMax=fNom+0.5, tTripf=0.24, tRecon=10, wind_type_sel_M=Time series, ave_speed_M=15, speed_series_M=[4  4   7.85  7.85  11.636  11.636  15   15   11.636  7.85  4    4 ], time_series_M=[0  25  75    100   150     175     225  250  300     350   400  451], turb_sel_M=Yes, turb_int_M=12}
      mask vMax=|
      | [1.1
      | 1.375]
      mask prompts: fNom "Nominal frequency (Hz)"; vNom "Nominal L-L voltage (kV)"; Nwt "Number of wind turbines"; vMin "Minimum voltage levels (pu) [Vmin2 Vmin1]"; vMax "Maximum voltage levels (pu) [Vmax1 Vmax2]"; tTripV "Trip times for U/O voltage protection (s) [V<Vmin2, Vmin2<V<Vmin1 or Vmax1<V<V max2, Vmax2<V]"; fMin "Minimum frequency (Hz) [fmin]"; fMax "Maximum frequency (Hz) [fmax]"; tTripf "Trip times for U/O frequency protection (Hz) [f<fmin or f>fmax]"; tRecon "Reconnection time (s)"; wind_type_sel_M "Type of wind speed"; ave_speed_M "Constant speed average (m/s)"; speed_series_M "Wind speed series (m/s) [v1 v2 v3 ...]"; time_series_M "Wind time series (s) [t1 t2 t3 ...]"; turb_sel_M "Insert turbulence"; turb_int_M "Turbulence intensity (%)"
      mask help:
      | Notes:
      | 1. The nominal output of each wind turbine for average wind speed of 15 m/s is 1.5 MW which is scalable by the  the wind speed in the control panel of the console is set to zero.
      mask init:
      | Fnom = fNom;
      | NumberOfUnits = Nwt;
      | 
      | Ts = 25e-6;
      | Ts_Power=Ts;
      | Ts_Control=2*Ts;
      | Ts_wind = 1000 * Ts;
      | 
      | 
      | % NumberOfUnits=6;
      | Pmec=1.5e6;     % Nominal power (W)
      | 
      | % Asynchronous machine data
      | Pnom=Pmec/0.9; % Nominal power (VA)
      | Vnom=575;       % Line-Line voltage (Vrms)
      | % Fnom=60;        %Hz
      | Rs=0.00706;     %pu
      | Lls=0.171;      %pu
      | Rr=0.005;       %pu
      | Llr=0.156;      %pu
      | Lm=2.9;         %pu
      | H=5.04;         %Inertia constant (s)
      | F=0.01;         %Friction factor (pu)
      | p=3;            %Number of pairs of poles
      | 
      | %PWM data
      | PWM_freq=27*Fnom;   %Not used with average model
      | 
      | %DC link
      | Vdc_nom=1200;       %Volts
      | C_DClink=10000e-6; %Farads
      | 
      | %Choke data
      | R_RL=0.30/100;  %pu
      | L_RL=0.30;      %pu
      | 
      | %Turbine data
      | power_C=1;   %pu
      | speed_C=1.2;    %pu
      | 
      | N_nom =1800;            % Nominal speed for generator [RPM] for 1 pu
      | K_gb =105;              % Gearbox Ratio
      | w_nom = speed_C * N_nom*pi/30;    % Nominal speed for generator [rad/s]
      | w_eol_nom = w_nom/K_gb; % Nominal speed for low speed side [rad/s]
      | rotor_dia = 72;         % rotor diameter [m]
      | length_scale = 600;     % lenght scale for wind speed generation [m]
      | lowpass_ts_wind = 5;    % low pass filer settling time for wind speed generator [s]
      | 
      | %High-voltage lines
      | dist=80;
      | 
      | %Filters
      | filter_value_2=473e3;
      mask TypeOptions wind_type_sel_M: Constant wind | Time series
      mask TypeOptions turb_sel_M: Yes | No
      mask DialogControl ParameterTabVar0 Prompt: Parameters
      mask DialogControl ParameterTabVar01 Prompt: Protection settings
      mask DialogControl ParameterTabVar012 Prompt: Wind parameters
      mask Display: image(imread('WT.jpg'))
  Wind Farm (DFIG Type)1 : Subsystem  mask(Wind Farm (DFIG Type)){fNom=fNom, vNom=1.025*vNomHV*(1E-3), Nwt=106, vMin=[0.5, 0.88], vMax=|, tTripV=[0.24  4.8  0.24], fMin=fNom-0.7, fMax=fNom+0.5, tTripf=0.24, tRecon=10, wind_type_sel_M=Time series, ave_speed_M=15, speed_series_M=[4  4   7.85  7.85  11.636  11.636  15   15   11.636  7.85  4    4 ], time_series_M=[0  25  75    100   150     175     225  250  300     350   400  451], turb_sel_M=Yes, turb_int_M=12}
      mask vMax=|
      | [1.1
      | 1.375]
      mask prompts: fNom "Nominal frequency (Hz)"; vNom "Nominal L-L voltage (kV)"; Nwt "Number of wind turbines"; vMin "Minimum voltage levels (pu) [Vmin2 Vmin1]"; vMax "Maximum voltage levels (pu) [Vmax1 Vmax2]"; tTripV "Trip times for U/O voltage protection (s) [V<Vmin2, Vmin2<V<Vmin1 or Vmax1<V<V max2, Vmax2<V]"; fMin "Minimum frequency (Hz) [fmin]"; fMax "Maximum frequency (Hz) [fmax]"; tTripf "Trip times for U/O frequency protection (Hz) [f<fmin or f>fmax]"; tRecon "Reconnection time (s)"; wind_type_sel_M "Type of wind speed"; ave_speed_M "Constant speed average (m/s)"; speed_series_M "Wind speed series (m/s) [v1 v2 v3 ...]"; time_series_M "Wind time series (s) [t1 t2 t3 ...]"; turb_sel_M "Insert turbulence"; turb_int_M "Turbulence intensity (%)"
      mask help:
      | Notes:
      | 1. The nominal output of each wind turbine for average wind speed of 15 m/s is 1.5 MW which is scalable by the  the wind speed in the control panel of the console is set to zero.
      mask init: same as SSN_39busRT_Ctrl_4WT_19B/SM_master/4 WT/SS_windfarm1to2/Wind Farm (DFIG Type)
      mask TypeOptions wind_type_sel_M: Constant wind | Time series
      mask TypeOptions turb_sel_M: Yes | No
      mask DialogControl ParameterTabVar0 Prompt: Parameters
      mask DialogControl ParameterTabVar01 Prompt: Protection settings
      mask DialogControl ParameterTabVar012 Prompt: Wind parameters
      mask Display: image(imread('WT.jpg'))
  Aw1 : PMIOPort  Side=Left
  Bw1 : PMIOPort  Port=2  Side=Left
  Cw1 : PMIOPort  Port=3  Side=Left
  Aw2 : PMIOPort  Port=4  Side=Right
  Bw2 : PMIOPort  Port=5  Side=Right
  Cw2 : PMIOPort  Port=6  Side=Right
  wf12_meas : Outport
  tag scope: wt1_speed=global, wt2_speed=global
  wires:
  Ctrl_wf12/1 -> OpComm/1
  Demux/1 -> Demux2/1
  OpComm/1 -> Demux/1
  Simulation monitoring1/1(sim_info) -> [sim_info]
  Bus Creator1/1 -> Memory2/1
  Wind Farm (DFIG Type)/1(WT_Meas1) -> Bus Creator1/1  "windfamr1 PQ speed"
  [wt1_speed] -> Wind Farm (DFIG Type)/1(Wind Power)
  Demux/2 -> Demux1/1
  Demux1/2 -> [CB_wf_ns]
  Demux1/1 -> [CB_vs_wf]
  [CB_wf_ns] -> Terminator/1
  [CB_vs_wf] -> Terminator1/1
  Wind Farm (DFIG Type)1/1(WT_Meas2) -> Bus Creator1/2  "windfram2 PQ speed"
  Memory2/1 -> wf12_meas/1
  [wt2_speed] -> Wind Farm (DFIG Type)1/1(Wind Power)
  [sim_info] -> Bus Creator1/3  "computation wf1"
  Demux2/1 -> [wt1_speed]
  Demux2/2 -> [wt2_speed]
  connections:
  Aw2/RConn1 -- Wind Farm (DFIG Type)1/LConn1
  Bw2/RConn1 -- Wind Farm (DFIG Type)1/LConn2
  Cw2/RConn1 -- Wind Farm (DFIG Type)1/LConn3
  Cw1/RConn1 -- Wind Farm (DFIG Type)/LConn3
  Bw1/RConn1 -- Wind Farm (DFIG Type)/LConn2
  Aw1/RConn1 -- Wind Farm (DFIG Type)/LConn1

== system SSN_39busRT_Ctrl_4WT_19B/SM_master/4 WT/SS_windfarm3to4 ==
  Ctrl_wf34 : Inport
  Bus Creator1 : BusCreator  Inputs=3
  Demux1 : Demux  Outputs=[1 1]
  Demux2 : Demux  Outputs=[2 2]
  Demux3 : Demux  Outputs=[1 1]
  Memory2 : Memory
  OpComm : rtlab/OpComm  nbport=1  groupe_acq=1  subsys_rate=Ts  st=Ts  Synchronization=on  Interpolation=on  Threshold=1.0  Missed_Data=off  Sim_Time=off  Samples=off  dynSigOut=off  from_console=0  warning_done=off  writeOpCommFile=off  Offset=off
      settings: SourceProductName=RT-LAB
  Simulation monitoring1 : Subsystem
  Terminator : Terminator
  Terminator1 : Terminator
  Wind Farm (DFIG Type) : Subsystem  mask(Wind Farm (DFIG Type)){fNom=fNom, vNom=1.025*vNomHV*(1E-3), Nwt=266, vMin=[0.5, 0.88], vMax=|, tTripV=[0.24  4.8  0.24], fMin=fNom-0.7, fMax=fNom+0.5, tTripf=0.24, tRecon=10, wind_type_sel_M=Time series, ave_speed_M=15, speed_series_M=[4  4   7.85  7.85  11.636  11.636  15   15   11.636  7.85  4    4 ], time_series_M=[0  25  75    100   150     175     225  250  300     350   400  451], turb_sel_M=Yes, turb_int_M=12}
      mask vMax=|
      | [1.1
      | 1.375]
      mask prompts: fNom "Nominal frequency (Hz)"; vNom "Nominal L-L voltage (kV)"; Nwt "Number of wind turbines"; vMin "Minimum voltage levels (pu) [Vmin2 Vmin1]"; vMax "Maximum voltage levels (pu) [Vmax1 Vmax2]"; tTripV "Trip times for U/O voltage protection (s) [V<Vmin2, Vmin2<V<Vmin1 or Vmax1<V<V max2, Vmax2<V]"; fMin "Minimum frequency (Hz) [fmin]"; fMax "Maximum frequency (Hz) [fmax]"; tTripf "Trip times for U/O frequency protection (Hz) [f<fmin or f>fmax]"; tRecon "Reconnection time (s)"; wind_type_sel_M "Type of wind speed"; ave_speed_M "Constant speed average (m/s)"; speed_series_M "Wind speed series (m/s) [v1 v2 v3 ...]"; time_series_M "Wind time series (s) [t1 t2 t3 ...]"; turb_sel_M "Insert turbulence"; turb_int_M "Turbulence intensity (%)"
      mask help:
      | Notes:
      | 1. The nominal output of each wind turbine for average wind speed of 15 m/s is 1.5 MW which is scalable by the  the wind speed in the control panel of the console is set to zero.
      mask init: same as SSN_39busRT_Ctrl_4WT_19B/SM_master/4 WT/SS_windfarm1to2/Wind Farm (DFIG Type)
      mask TypeOptions wind_type_sel_M: Constant wind | Time series
      mask TypeOptions turb_sel_M: Yes | No
      mask DialogControl ParameterTabVar0 Prompt: Parameters
      mask DialogControl ParameterTabVar01 Prompt: Protection settings
      mask DialogControl ParameterTabVar012 Prompt: Wind parameters
      mask Display: image(imread('WT.jpg'))
  Wind Farm (DFIG Type)2 : Subsystem  mask(Wind Farm (DFIG Type)){fNom=fNom, vNom=1.025*vNomHV*(1E-3), Nwt=333, vMin=[0.5, 0.88], vMax=|, tTripV=[0.24  4.8  0.24], fMin=fNom-0.7, fMax=fNom+0.5, tTripf=0.24, tRecon=10, wind_type_sel_M=Time series, ave_speed_M=15, speed_series_M=[4  4   7.85  7.85  11.636  11.636  15   15   11.636  7.85  4    4 ], time_series_M=[0  25  75    100   150     175     225  250  300     350   400  451], turb_sel_M=Yes, turb_int_M=12}
      mask vMax=|
      | [1.1
      | 1.375]
      mask prompts: fNom "Nominal frequency (Hz)"; vNom "Nominal L-L voltage (kV)"; Nwt "Number of wind turbines"; vMin "Minimum voltage levels (pu) [Vmin2 Vmin1]"; vMax "Maximum voltage levels (pu) [Vmax1 Vmax2]"; tTripV "Trip times for U/O voltage protection (s) [V<Vmin2, Vmin2<V<Vmin1 or Vmax1<V<V max2, Vmax2<V]"; fMin "Minimum frequency (Hz) [fmin]"; fMax "Maximum frequency (Hz) [fmax]"; tTripf "Trip times for U/O frequency protection (Hz) [f<fmin or f>fmax]"; tRecon "Reconnection time (s)"; wind_type_sel_M "Type of wind speed"; ave_speed_M "Constant speed average (m/s)"; speed_series_M "Wind speed series (m/s) [v1 v2 v3 ...]"; time_series_M "Wind time series (s) [t1 t2 t3 ...]"; turb_sel_M "Insert turbulence"; turb_int_M "Turbulence intensity (%)"
      mask help:
      | Notes:
      | 1. The nominal output of each wind turbine for average wind speed of 15 m/s is 1.5 MW which is scalable by the  the wind speed in the control panel of the console is set to zero.
      mask init: same as SSN_39busRT_Ctrl_4WT_19B/SM_master/4 WT/SS_windfarm1to2/Wind Farm (DFIG Type)
      mask TypeOptions wind_type_sel_M: Constant wind | Time series
      mask TypeOptions turb_sel_M: Yes | No
      mask DialogControl ParameterTabVar0 Prompt: Parameters
      mask DialogControl ParameterTabVar01 Prompt: Protection settings
      mask DialogControl ParameterTabVar012 Prompt: Wind parameters
      mask Display: image(imread('WT.jpg'))
  Aw3 : PMIOPort  Side=Left
  Bw3 : PMIOPort  Port=2  Side=Left
  Cw3 : PMIOPort  Port=3  Side=Left
  Aw4 : PMIOPort  Port=4  Side=Right
  Bw4 : PMIOPort  Port=5  Side=Right
  Cw4 : PMIOPort  Port=6  Side=Right
  wf34_meas : Outport
  tag scope: wt3_speed=global, wt4_speed=global
  wires:
  [wt4_speed] -> Wind Farm (DFIG Type)2/1(Wind Power)
  Memory2/1 -> wf34_meas/1
  Wind Farm (DFIG Type)2/1(WT_Meas1) -> Bus Creator1/2  "windfram4 PQ speed"
  [CB_vs_wf] -> Terminator1/1
  [CB_wf_ns] -> Terminator/1
  [wt3_speed] -> Wind Farm (DFIG Type)/1(Wind Power)
  [sim_info] -> Bus Creator1/3  "computation wf45"
  Wind Farm (DFIG Type)/1(WT_Meas1) -> Bus Creator1/1  "windfamr3 PQ speed"
  Bus Creator1/1 -> Memory2/1
  Simulation monitoring1/1(sim_info) -> [sim_info]
  OpComm/1 -> Demux2/1
  Ctrl_wf34/1 -> OpComm/1
  Demux2/2 -> Demux1/1
  Demux1/2 -> [CB_wf_ns]
  Demux1/1 -> [CB_vs_wf]
  Demux2/1 -> Demux3/1
  Demux3/1 -> [wt3_speed]
  Demux3/2 -> [wt4_speed]
  connections:
  Cw4/RConn1 -- Wind Farm (DFIG Type)2/LConn3
  Bw4/RConn1 -- Wind Farm (DFIG Type)2/LConn2
  Aw4/RConn1 -- Wind Farm (DFIG Type)2/LConn1
  Wind Farm (DFIG Type)/LConn1 -- Aw3/RConn1
  Wind Farm (DFIG Type)/LConn3 -- Cw3/RConn1
  Wind Farm (DFIG Type)/LConn2 -- Bw3/RConn1

== system SSN_39busRT_Ctrl_4WT_19B/SM_master/4 WT/controlWt ==
  Subsystem : Subsystem
  Windfarm Control : Subsystem
  "ctrl_wf12 " : Outport
  ctrl_wf34 : Outport  Port=2
  tag scope: WF_CB_ctr=global
  wires:
  Windfarm Control/1(wf_CB_ctr) -> [WF_CB_ctr]
  Subsystem/2(ctrl_wf34) -> ctrl_wf34/1
  Subsystem/1("ctrl_wf12 ") -> "ctrl_wf12 "/1

== system SSN_39busRT_Ctrl_4WT_19B/SM_master/G1/G1 ==
  note: Reactive Power
  note: Field Current
  note: Stator Current
  note: Stator Voltage
  note: Active Power
  note: Rotor Speed
  note: Measurement Outputs
  note: Mechanical
      | Power (Pm)
  note: Field Voltage (Vf)
  note: Stator Current
  note: Reactive Power
  note: Stator Voltage
  note: Voltage Reference
  note: Field Current
  note: Active Power
  note: SM Measurement Signal
  note: Rotor Speed Reference
  note: Rotor Speed
  wref (pu) : Inport
  Vref (pu) : Inport  Port=2
  Generator Measurements (Output) : Subsystem
  Governor model with Droop : Subsystem
  Ground7 : Ground
  ST6C EXCITER-1 : Subsystem
  Synchronous Machine : spsSynchronousMachinepuStandardLib/Synchronous Machine pu Standard  PresetModel=No  MechanicalLoad=Mechanical power Pm  ShowDetailedParameters=on  RotorType=Salient-pole  Units=per unit standard parameters  MeasurementBus=off  NominalParameters="[ Pn  Vn   f ]"  Reactances1=[ 31 32 33 34 35 36 37 ]  Reactances2=[ 1.305, 0.296, 0.252, 0.474, 0.243, 0.18 ]  dAxisTimeConstants=Short-circuit  qAxisTimeConstants=Open-circuit  TimeConstants1=[]  TimeConstants2=[]  TimeConstants3=[]  TimeConstants4=[]  TimeConstants5=[ 1.01, 0.053, 0.1 ]  TimeConstants6=[]  TimeConstants7=[]  TimeConstants8=[]  StatorResistance=2.8544e-3  Mechanical=[H1 0 2]  PolePairs=2  InitialConditions=[0 -62.5202 1.01055 1.01055 1.01055 8.25986 -111.74 128.26 1.32748]  SetSaturation=off  Saturation=[0.6404,0.7127,0.8441,0.9214,0.9956,1.082,1.19,1.316,1.457;0.7,0.7698,0.8872,0.9466,0.9969,1.046,1.1,1.151,1.201]  LoadFlowParameters=[1 150000000 0 0]  TsPowergui=0  TsBlock=-1  IterativeModel=Trapezoidal non iterative  IterativeDiscreteModel=Trapezoidal non iterative  BusType=PV  Pref=42e6  Qref=0  Qmin=-50000000  Qmax=50000000  PLF=0  QLF=0
      settings: SourceProductBaseCode=PS
  A : PMIOPort  Side=Right
  B : PMIOPort  Port=2  Side=Right
  C : PMIOPort  Port=3  Side=Right
  sm1 : Outport  VectorParamsAs1DForOutWhenUnconnected=off
  wires:
  Synchronous Machine/1 -> Generator Measurements (Output)/1(m)
  Vref (pu)/1 -> ST6C EXCITER-1/1(Vref)
  Governor model with Droop/1(Pmec (pu)) -> Synchronous Machine/1
  wref (pu)/1 -> Governor model with Droop/1(wref (pu)1)
  Ground7/1 -> ST6C EXCITER-1/5(Vstab)
  [QT1st] -> ST6C EXCITER-1/6(QT)
  [It1st] -> ST6C EXCITER-1/3(It)
  [PT1st] -> ST6C EXCITER-1/7(PT)
  ST6C EXCITER-1/1(Efd) -> [Efd1st], Synchronous Machine/2
  Generator Measurements (Output)/2(wm) -> [wm1]
  Generator Measurements (Output)/4(Ifd) -> [Ifd1st]
  Generator Measurements (Output)/5(It) -> [It1st]
  Generator Measurements (Output)/1(sm) -> sm1/1
  Generator Measurements (Output)/7(QT) -> [QT1st]
  Generator Measurements (Output)/6(PT) -> [PT1st]
  Generator Measurements (Output)/3(Vt) -> [Vt1st]
  [wm1] -> Governor model with Droop/2(w (pu))
  [Vt1st] -> ST6C EXCITER-1/2(Vt)
  [Ifd1st] -> ST6C EXCITER-1/4(Ifd)
  [PT1st] -> Governor model with Droop/3(Input)
  connections:
  B/RConn1 -- Synchronous Machine/RConn2
  C/RConn1 -- Synchronous Machine/RConn3
  A/RConn1 -- Synchronous Machine/RConn1
